simulink model "cordic_16bit_test"  (Simulink 6.0)
settings: Solver=ode3  StartTime=0.0  StopTime=500.0  RelTol=1e-3  SampleTimeConstraint=Specified
undefined symbols (not defined in the file): cordic_16bit, DSPBuilder_cordic_16bit_test, SOURCE_FILE, VHDL
libraries: bus_alteradspbuilder x2, hdl_import_alteradspbuilder x1
settings Model: LastModifiedBy=kumm
settings MATStruct: SampleTime=1  Offset=0  Priority=[1.0]

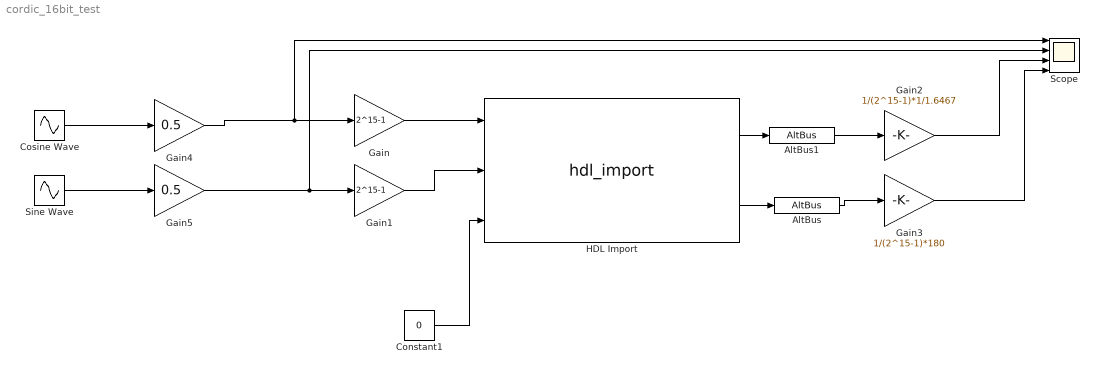
== system cordic_16bit_test ==
  AltBus : bus_alteradspbuilder/AltBus  Description=Sign Binary Fractionnal  sgn=Signed Integer  nodetype=Internal Node  bwl=16  bwr=0  sat=off  rnd=off  bp=off  mask_cst=0  LocPin=any  cst=0  modulename=AltBus  nSgCpl=0  SIGNALCOMPILER_PARAMS=sgn;Signed Integer;nodetype;Internal Node;bwl;16;bwr;0;sat;off;rnd;off;cst;0;LocPin;any;
  AltBus1 : bus_alteradspbuilder/AltBus  Description=Sign Binary Fractionnal  sgn=Unsigned Integer  nodetype=Internal Node  bwl=16  bwr=0  sat=off  rnd=off  bp=off  mask_cst=0  LocPin=any  cst=0  modulename=AltBus1  nSgCpl=0  SIGNALCOMPILER_PARAMS=sgn;Unsigned Integer;nodetype;Internal Node;bwl;16;bwr;0;sat;off;rnd;off;cst;0;LocPin;any;
  Constant1 : Constant  Value=0
  Cosine Wave : Sin  Frequency=0.1  Phase=pi/2  SampleTime=0
  Gain : Gain  Gain=2^15-1
  Gain1 : Gain  Gain=2^15-1
  Gain2 : Gain  Gain=1/(2^15-1)*1/1.6467
  Gain3 : Gain  Gain=1/(2^15-1)*180
  Gain4 : Gain  Gain=0.5
  Gain5 : Gain  Gain=0.5
  HDL Import : hdl_import_alteradspbuilder/hdl_import  vofile=DSPBuilder_cordic_16bit_test/cordic_16bit.vo  xmlmapfile=E:\altera\DSPBuilder\Altlib\SimgenCMap.xml  src_file=..\VHDL\cordic_16bit.vhd;  n_input_port=3  n_output_port=2  n_clocks=1  array_input=i_i q_i rst_i  array_output=magnitude_o phase_o  array_clocks=clk_i  clockname=clk_i  inptbwl=16 16 1  outptbwl=16 16  dspbuilder_path=E:\altera\DSPBuilder\Altlib  HDLInputPortsMappingAltera=i_i.16.0.s, q_i.16.0.s, rst_i.1.0.b  HDLOutputPortsMappingAltera=magnitude_o.16.0.s, phase_o.16.0.s  HDLImplicitPortsMappingAltera=clk_i.clock  HDLParameterMappingAltera=NOHDLPARAMETER  HDLLibraryInformationAltera=ADD_COMPONENT_SECTION  HDLComponentNameAltera=cordic_16bit  UseQPF=0  TopLevelName=cordic_16bit  q_src_files=..\VHDL\cordic_16bit.vhd;  q_src_types=SOURCE_FILE;
  Scope : Scope  NumInputPorts=4
      settings: TimeRange=500  YMin=-0.5~-0.5~0~-200  YMax=0.5~0.5~0.7000000000000001~200
  Sine Wave : Sin  Frequency=0.1  SampleTime=0
  wires:
  Constant1/1 -> HDL Import/3
  Gain1/1 -> HDL Import/2
  HDL Import/1 -> AltBus1/1
  HDL Import/2 -> AltBus/1
  Gain/1 -> HDL Import/1
  AltBus1/1 -> Gain2/1
  AltBus/1 -> Gain3/1
  Gain4/1 -> Gain/1, Scope/1
  Gain5/1 -> Gain1/1, Scope/2
  Gain2/1 -> Scope/3
  Cosine Wave/1 -> Gain4/1
  Sine Wave/1 -> Gain5/1
  Gain3/1 -> Scope/4
